simulink model "Katex_FullCar_R2017b_V03"  (R2026a)
settings: Solver=ode1  StopTime=1000  FixedStep=Ts  EnableMultiTasking=on
PostLoadFcn:
  | , if any(exist('dsrtsu_mdlpostloadfcn', 'file') == [2, 3, 6]), try dsrtsu_mdlpostloadfcn('Execute', bdroot); catch fprintf('Error in PostLoadFcn (dsrtsu_mdlpostloadfcn) for model "%s":\n %s\n', bdroot, lasterr); end, end,
  | , if any(exist('dsrtsu_mdlpostloadfcn', 'file') ~= 0), dsrtsu_mdlpostloadfcn('Execute', bdroot); end,
InitFcn:
  | , if any(exist('rtifpga_mdlclblib', 'file') ~= 0), rtifpga_mdlclblib('Init', bdroot); end,
  | 
  | 
  | init
undefined symbols (not defined in the file): locklim_sus, roundN, Ts
libraries: sl_discontinuities x29, simulink_extras x26, simulink x22, mjLib x1
(part 3 of 10)

== system Katex_FullCar_R2017b_V03/DGIST/_High_Level_Ctrl/Chassis_FF_ctrl ==
  note: m/s
  note: Output
      |
      | Load단
      |
      | FL
      | FR
      | RL
      | RR
  note: rad/s
  note: m/s
  note: deg/s
  note: rad/s 여야함
  note: rad/s
  Add1 : Sum  Inputs=+-
  Add3 : Sum
  Divide1 : Product  Inputs=**
  Kinematic_Mapping_FF : MATLAB Function  TreatAsAtomicUnit=on
  Multiply1 : Gain  Gain=pi/180
  Multiply3 : Gain  Gain=180/pi
  Mux : Mux  Inputs=2
  P Control1 : Subsystem
      mask Display: disp('P Control');
  FF_DriveVel_ref : Outport
  FF_SteerPos_ref : Outport  Port=2
  Body_ref_scope : Outport  Port=3
  wires:
  [Body_Vx_ref] -> Kinematic_Mapping_FF/1(Vx_ref)
  [YawRate_FB_ref] -> Kinematic_Mapping_FF/2(YawRate_ref)
  [Wheel_Radius] -> Kinematic_Mapping_FF/5(WheelRadius)
  [Steer_Ref_Limit] -> Kinematic_Mapping_FF/6(SteerLimit)
  Kinematic_Mapping_FF/1(DriveVel_ref) -> FF_DriveVel_ref/1
  Kinematic_Mapping_FF/2(SteerPos_ref) -> FF_SteerPos_ref/1
  [Chassis_wheelbase] -> Kinematic_Mapping_FF/3(L)
  [Chassis_wheelTrack] -> Kinematic_Mapping_FF/4(W)
  Mux/1 -> Body_ref_scope/1
  [Body_Vx_ref] -> Mux/1
  [Body_YawRate_ref] -> Multiply3/1
  Multiply3/1 -> Mux/2
  [Body_YawRate_FB_OnOff] -> Divide1/2
  Divide1/1 -> P Control1/1(err)
  [Body_YawRate_ref] -> Add1/1, Add3/1
  Add3/1 -> [YawRate_FB_ref]
  Multiply1/1 -> Add1/2
  P Control1/1(Out1) -> Add3/2
  Add1/1 -> Divide1/1
  [AngRateYaw_degps] -> Multiply1/1

== system Katex_FullCar_R2017b_V03/DGIST/_High_Level_Ctrl/If Action Subsystem1 ==
  In1 : Inport
  In2 : Inport  Port=2
  In3 : Inport  Port=3
  Action Port : ActionPort  ActionPortLabel=elseif(u1 == 1)
  Out1 : Outport  VectorParamsAs1DForOutWhenUnconnected=off
  Out2 : Outport  Port=2  VectorParamsAs1DForOutWhenUnconnected=off
  Out3 : Outport  Port=3  VectorParamsAs1DForOutWhenUnconnected=off
  wires:
  In1/1 -> Out1/1
  In2/1 -> Out2/1
  In3/1 -> Out3/1

== system Katex_FullCar_R2017b_V03/DGIST/_High_Level_Ctrl/If Action Subsystem5 ==
  In1 : Inport
  In2 : Inport  Port=2
  In3 : Inport  Port=3
  Action Port : ActionPort  ActionPortLabel=if(u1 == 0)
  Out1 : Outport  VectorParamsAs1DForOutWhenUnconnected=off
  Out2 : Outport  Port=2  VectorParamsAs1DForOutWhenUnconnected=off
  Out3 : Outport  Port=3  VectorParamsAs1DForOutWhenUnconnected=off
  wires:
  In1/1 -> Out1/1
  In2/1 -> Out2/1
  In3/1 -> Out3/1

== system Katex_FullCar_R2017b_V03/DGIST/_High_Level_Ctrl/Orientation_Pos_Ctrl ==
  note: deg
  note: rad
  note: Output
      |
      | Suspension Load-side Position (deg)
      |
      | FL
      | FR
      | RL
      | RR
  note: 모터 회전방향 확인 필요(부호 확인 필요)
      |
      | z의 양의 방향을 위쪽으로 정의했다면
      |
      | Load side vel
      | SusVel_ref >0 => 아래로 이동
      | SusVel_ref<0 => 위로 이동
  note: Load deg
  note: deg
  Body_Pitch_PID_ctrl : Subsystem
  Body_Roll_PID_ctrl : Subsystem
  Constant : Constant  Value=180/pi
  Constant4 : Constant  Value=0
  Constant5 : Constant  Value=30
  Demux : Demux  Commented=on
  Divide : Product  Inputs=**
  Gain{,1..6} (7 alike) : Gain  Gain=pi/180
  Goto1 : Goto  Commented=on  GotoTag=SusFR_Load_Pos_Ref  TagVisibility=global
  Goto2 : Goto  Commented=on  GotoTag=SusRL_Load_Pos_Ref  TagVisibility=global
  Goto3 : Goto  Commented=on  GotoTag=SusRR_Load_Pos_Ref  TagVisibility=global
  Goto4 : Goto  Commented=on  GotoTag=SusFL_Load_Pos_Ref  TagVisibility=global
  MATLAB Function : MATLAB Function  TreatAsAtomicUnit=on
  Mux : Mux
  Mux1 : Mux  Inputs=2
  Scope : Scope
      settings: ActiveDisplayYMinimum=-1  ActiveDisplayYMaximum=1  DataLoggingVariableName=ScopeData7
  Out1 : Outport  VectorParamsAs1DForOutWhenUnconnected=off
  Ori_Sus_Load_Pos_Ref : Outport  Port=2
  wires:
  [Chassis_wheelbase] -> MATLAB Function/4(RobotWidth)
  [Chassis_wheelTrack] -> MATLAB Function/5(RobotLength)
  [Sus_Length] -> MATLAB Function/6(SusLinkLength)
  Demux/4 -> Goto3/1
  Demux/3 -> Goto2/1
  Demux/2 -> Goto1/1
  Demux/1 -> Goto4/1
  MATLAB Function/1(SusPos_ref) -> Divide/1
  Constant/1 -> Divide/2
  Mux/1 -> MATLAB Function/3(SusPos_neutral)
  Gain/1 -> MATLAB Function/1(Roll_ref)
  Gain1/1 -> MATLAB Function/2(Pitch_ref)
  Gain2/1 -> Mux/1
  Gain3/1 -> Mux/2
  Gain4/1 -> Mux/3
  Gain5/1 -> Mux/4
  Constant4/1 -> Gain5/1, Gain4/1, Gain3/1, Gain2/1
  Gain6/1 -> MATLAB Function/7(SusPosLimit)
  Constant5/1 -> Gain6/1
  [Body_RollRate_ref] -> Body_Roll_PID_ctrl/1(In1)
  [Body_PitchRate_ref] -> Body_Pitch_PID_ctrl/1(In1)
  Body_Pitch_PID_ctrl/1(Out1) -> Gain1/1
  Body_Roll_PID_ctrl/1(Out1) -> Gain/1
  [AngRoll_deg] -> Body_Roll_PID_ctrl/2(In2)
  [AngPitch_deg] -> Body_Pitch_PID_ctrl/2(In2)
  Mux1/1 -> Out1/1
  [Body_RollRate_ref] -> Mux1/1
  [Body_PitchRate_ref] -> Mux1/2
  Divide/1 -> Scope/1, Ori_Sus_Load_Pos_Ref/1

== system Katex_FullCar_R2017b_V03/DGIST/_High_Level_Ctrl/Orientation_Vel_Ctrl ==
  note: rad/s
  note: Output
      |
      | Suspension Load-side Velocity
      |
      | FL
      | FR
      | RL
      | RR
  note: Sus Load Position 가져와야함
  note: 모터 회전방향 확인 필요(부호 확인 필요)
      |
      | z의 양의 방향을 위쪽으로 정의했다면
      |
      | Load side vel
      | SusVel_ref >0 => 아래로 이동
      | SusVel_ref<0 => 위로 이동
  DOB_Dis : Constant  Value=0
  Demux : Demux
  MATLAB Function : MATLAB Function  TreatAsAtomicUnit=on
  Ts : Constant  Value=Ts
  tag scope: SusFL_Load_Vel_Ref=global, SusFR_Load_Vel_Ref=global, SusRL_Load_Vel_Ref=global, SusRR_Load_Vel_Ref=global
  wires:
  [Body_RollRate_ref] -> MATLAB Function/1(RollRate_ref)
  [Body_PitchRate_ref] -> MATLAB Function/2(PitchRate_ref)
  DOB_Dis/1 -> MATLAB Function/5(disturbance)
  [Chassis_wheelTrack] -> MATLAB Function/7(RobotWidth)
  [Chassis_wheelbase] -> MATLAB Function/8(RobotLength)
  [Sus_LinkLength] -> MATLAB Function/9(SusLinkLength)
  Ts/1 -> MATLAB Function/11(Ts)
  [Ori_DOB_CutOff] -> MATLAB Function/10(DOB_cutoff_freq)
  [Ori_DOB_OnOff] -> MATLAB Function/12(DOB_onoff)
  MATLAB Function/1(SusVel_ref) -> Demux/1
  Demux/4 -> [SusRR_Load_Vel_Ref]
  Demux/3 -> [SusRL_Load_Vel_Ref]
  Demux/2 -> [SusFR_Load_Vel_Ref]
  Demux/1 -> [SusFL_Load_Vel_Ref]

== system Katex_FullCar_R2017b_V03/DGIST/_Low_Level_Ctrl/Driving_Low_Level_Controller ==
  note: Motor Input 4X1
  note: Target Torque
  note: Output
      |
      | 1: Motor angular velocity (단위가 RPM 이여야함)
      | 2: Motor Torque (단위가 Target Torque 여야함)
      | 3: 전륜 RPM / 후륜 Target Torque 0 이여야함
      |
      | 각 Box Output에 input mode도 같이 나와야함 4X1로 나와야함
      | (8: position / 9: Velocity / 10: Torque)
  note: 0: Pos Mode(안씀)
      | 1: Vel Mode
      | 2: Torque Mode
      | 3: FB(전륜 Vel Mode, 후륜 Torque Mode)
  note: Motor Input Mode
  note: Motor Input Mode
  note: 전륜: RPM/ 후륜: Target Torque 0
  note: Motor Input Mode
  note: Load m/s
  In1 : Inport
  Demux : Demux
  Divide1 : Product  Inputs=**
  FB Mode : Subsystem  TreatAsAtomicUnit=on
  If1 : If  IfExpression=u1 == 1  ElseIfExpressions=u1 == 2,u1 == 3
  Merge1 : Merge  Inputs=3
  Merge2 : Merge  Inputs=3
  Torque Mode : Subsystem  TreatAsAtomicUnit=on
  Tunning reference box : Subsystem
  Velocity Mode : Subsystem  TreatAsAtomicUnit=on
  Out1 : Outport
  tag scope: DriFL_Motor_OperationMode=global, DriFR_Motor_OperationMode=global, DriRL_Motor_OperationMode=global, DriRR_Motor_OperationMode=global
  wires:
  If1/1 -> Velocity Mode/Action
  If1/2 -> Torque Mode/Action
  [ctrl_onoff] -> Divide1/1
  [Dri_Motor_Mode] -> If1/1
  Demux/1 -> [DriFL_Motor_OperationMode]
  Merge2/1 -> Demux/1
  Demux/4 -> [DriRR_Motor_OperationMode]
  Velocity Mode/1(Out1) -> Merge1/1
  Velocity Mode/2(Out2) -> Merge2/1
  Demux/2 -> [DriFR_Motor_OperationMode]
  If1/3 -> FB Mode/Action
  Merge1/1 -> Divide1/2
  Demux/3 -> [DriRL_Motor_OperationMode]
  [Dri_Vel] -> FB Mode/1(In1)
  In1/1 -> [Dri_Vel]
  Divide1/1 -> Out1/1
  [Dri_Vel] -> Velocity Mode/1(In1)
  FB Mode/1(Out1) -> Merge1/3
  Torque Mode/1(Out1) -> Merge1/2
  FB Mode/2(Out2) -> Merge2/3
  Torque Mode/2(Out2) -> Merge2/2

== system Katex_FullCar_R2017b_V03/DGIST/_Low_Level_Ctrl/Steering_Low_Level_Controller ==
  note: Motor Input 4X1
  note: Motor Input Mode
  note: Target Torque
  note: Motor Input Mode
  note: 0: Pos Mode
      | 1: Vel Mode(안씀)
      | 2: Torque Mode
      | 3: FB(Pos Mode)
  note: Output
      |
      | 0: Motor angular Position (단위 cnt)
      | 1: Motor angular velocity (안씀)
      | 2: Motor Target Torque (Target Torque)
      |
      | 각 Box Output에 input mode도 같이 나와야함 4X1로 나와야함
      | (8: position / 9: Velocity / 10: Torque)
  note: cnt
  note: cnt
  In1 : Inport
  Constant : Constant  Value=0
  Demux : Demux
  Divide1 : Product  Inputs=**
  Gain : Gain
  If1 : If  IfExpression=u1 == 0  ElseIfExpressions=u1 == 2
  Merge : Merge
  Merge1 : Merge
  Mux : Mux
  Position Mode : Subsystem  TreatAsAtomicUnit=on
  Sine Wave : Sin  Amplitude=10  Frequency=0.2  SampleTime=0
  Torque Mode : Subsystem  TreatAsAtomicUnit=on
  Out1 : Outport
  tag scope: StrFL_Motor_OperationMode=global, StrFR_Motor_OperationMode=global, StrRL_Motor_OperationMode=global, StrRR_Motor_OperationMode=global
  wires:
  If1/1 -> Position Mode/Action
  If1/2 -> Torque Mode/Action
  [ctrl_onoff] -> Divide1/1
  Divide1/1 -> Out1/1
  [Str_Motor_Mode] -> If1/1
  Demux/1 -> [StrFL_Motor_OperationMode]
  Demux/4 -> [StrRR_Motor_OperationMode]
  Demux/2 -> [StrFR_Motor_OperationMode]
  Demux/3 -> [StrRL_Motor_OperationMode]
  In1/1 -> [Str_Load_Pos_Ref]
  Mux/1 -> Position Mode/1(In1)
  Gain/1 -> Mux/2, Mux/3, Mux/4, Mux/1
  Constant/1 -> Gain/1
  Torque Mode/1(Out1) -> Merge/2
  Merge/1 -> Divide1/2
  Position Mode/1(Out1) -> Merge/1
  Merge1/1 -> Demux/1
  Position Mode/2(Out2) -> Merge1/1
  Torque Mode/2(Out2) -> Merge1/2

== system Katex_FullCar_R2017b_V03/DGIST/_Low_Level_Ctrl/Suspension_Low_Level_Controller ==
  note: 추가해야 할 부분(Sus control부분에서)
      | Position Mapping 입력부분 RollRate,PitchRate 같이 사용하는 중 (High level)
      | SusPosLimit 연결 필요(High level)
      | Velocity DOB 입력 미연결 상태 IMU, SusPos_act 연결필요
      | DOB disturbance check 부분 4X1로 만들어야 할 필요 있음
  note: Motor Input 4X1
  note: Target Torque
  note: 0: Pos Mode
      | 1: Vel Mode
      | 2: Torque Mode
  note: Motor Input Mode
  note: RPM
  note: Motor Input Mode
  note: Motor Input Mode
  note: 0: Pos Mode
      | 1: Vel Mode
      | 2: Torque Mode (안씀)
      | 3: FB(전륜 Vel Mode, 후륜 Torque Mode) (안씀)
  note: Output
      |
      | 0: Motor angular Position (단위 cnt)
      | 1: Motor angular velocity (단위 RPM)
      | 2: Motor Target Torque (안씀)
      |
      | 각 Box Output에 input mode도 같이 나와야함 4X1로 나와야함
      | (8: position / 9: Velocity / 10: Torque)
  note: cnt
  note: Load deg
  In1 : Inport
  Demux : Demux
  Divide1 : Product  Inputs=**
  If1 : If  IfExpression=u1 == 0  ElseIfExpressions=u1 == 1,u1 == 2
  Merge : Merge  Inputs=3
  Merge1 : Merge  Inputs=3
  Position Mode : Subsystem  TreatAsAtomicUnit=on
  Torque Mode : Subsystem  TreatAsAtomicUnit=on
  Tunning reference box : Subsystem
  Velocity Mode : Subsystem  TreatAsAtomicUnit=on
  Out1 : Outport
  tag scope: SusFL_Motor_OperationMode=global, SusFR_Motor_OperationMode=global, SusRL_Motor_OperationMode=global, SusRR_Motor_OperationMode=global
  wires:
  If1/1 -> Position Mode/Action
  If1/2 -> Velocity Mode/Action
  [ctrl_onoff] -> Divide1/1
  [Sus_Motor_Mode] -> If1/1
  Demux/1 -> [SusFL_Motor_OperationMode]
  Demux/4 -> [SusRR_Motor_OperationMode]
  Demux/2 -> [SusFR_Motor_OperationMode]
  If1/3 -> Torque Mode/Action
  Demux/3 -> [SusRL_Motor_OperationMode]
  [Sus_Load_Deg_Limit] -> Position Mode/2(In2)
  [Sus_Load_Pos_Ref] -> Position Mode/1(In1)
  Merge/1 -> Demux/1
  Position Mode/2(Out2) -> Merge/1
  Velocity Mode/2(Out2) -> Merge/2
  Torque Mode/2(Out2) -> Merge/3
  Merge1/1 -> Divide1/2
  Position Mode/1(Out1) -> Merge1/1
  Velocity Mode/1(Out1) -> Merge1/2
  [Sus_Torque_Limit] -> Torque Mode/2(In2)
  In1/1 -> [Sus_Load_Pos_Ref]
  Torque Mode/1(Out1) -> Merge1/3
  [Sus_Load_Pos_Ref] -> Torque Mode/1(In1)
  Divide1/1 -> Out1/1

== system Katex_FullCar_R2017b_V03/DGIST/_Reference_Generator/If Action Subsystem1 ==
  In1 : Inport
  Action Port : ActionPort  ActionPortLabel=elseif(u1 == 2)
  Out1 : Outport  VectorParamsAs1DForOutWhenUnconnected=off
  wires:
  In1/1 -> Out1/1

== system Katex_FullCar_R2017b_V03/DGIST/_Reference_Generator/If Action Subsystem2 ==
  In1 : Inport
  Action Port : ActionPort  ActionPortLabel=elseif(u1 == 3)
  Demux : Demux
  Scope : Scope
      settings: DataLoggingVariableName=ScopeData2
  Terminator : Terminator
  Terminator1 : Terminator
  Terminator2 : Terminator
  Out1 : Outport  VectorParamsAs1DForOutWhenUnconnected=off
  wires:
  In1/1 -> Demux/1, Out1/1
  Demux/3 -> Scope/1
  Demux/1 -> Terminator/1
  Demux/2 -> Terminator1/1
  Demux/4 -> Terminator2/1

== system Katex_FullCar_R2017b_V03/DGIST/_Reference_Generator/If Action Subsystem3 ==
  In1 : Inport
  Action Port : ActionPort  ActionPortLabel=else
  Out1 : Outport  VectorParamsAs1DForOutWhenUnconnected=off
  wires:
  In1/1 -> Out1/1

== system Katex_FullCar_R2017b_V03/DGIST/_Reference_Generator/If Action Subsystem4 ==
  In1 : Inport
  Action Port : ActionPort  ActionPortLabel=if(u1 == 1)
  Out1 : Outport  VectorParamsAs1DForOutWhenUnconnected=off
  wires:
  In1/1 -> Out1/1

== system Katex_FullCar_R2017b_V03/DGIST/_Reference_Generator/Orientation Profile ==
  note: output
      |
      | Vx
      | gamma
      | RollRate
      | PitchRate
  Compare To Constant1 : simulink/Logic and Bit Operations/Compare To Constant  relop===  const=3  OutDataTypeStr=boolean
  Compare To Constant2 : simulink/Logic and Bit Operations/Compare To Constant  relop===  const=3  OutDataTypeStr=boolean
  Constant : Constant  Value=0
  Data Type Conversion1 : DataTypeConversion  OutDataTypeStr=double  SaturateOnIntegerOverflow=off  RndMeth=Floor
  Data Type Conversion2 : DataTypeConversion  OutDataTypeStr=double  SaturateOnIntegerOverflow=off  RndMeth=Floor
  Divide1 : Product  Inputs=**
  Divide2 : Product  Inputs=**
  MATLAB Function : MATLAB Function  TreatAsAtomicUnit=on
  MATLAB Function1 : MATLAB Function  TreatAsAtomicUnit=on
  Output : Mux
  Ref3_Output : Outport
  wires:
  Output/1 -> Ref3_Output/1
  Constant/1 -> Output/2, Output/1
  [Local_Time] -> MATLAB Function/1(t)
  Divide2/1 -> MATLAB Function/4(flag)
  [RollRate_freq_ref_cmd] -> MATLAB Function/2(f)
  [RollRate_mag_ref_cmd] -> MATLAB Function/3(mag)
  [Local_Time] -> MATLAB Function1/1(t)
  Divide1/1 -> MATLAB Function1/4(flag)
  [PitchRate_freq_ref_cmd] -> MATLAB Function1/2(f)
  [PitchRate_mag_ref_cmd] -> MATLAB Function1/3(mag)
  MATLAB Function/1(y) -> Output/3
  MATLAB Function1/1(y) -> Output/4
  Compare To Constant1/1 -> Data Type Conversion1/1
  Data Type Conversion1/1 -> Divide2/2
  [ctrl_onoff] -> Divide2/1
  [Scenario_cmd] -> Compare To Constant1/1
  [ctrl_onoff] -> Divide1/1
  Data Type Conversion2/1 -> Divide1/2
  [Scenario_cmd] -> Compare To Constant2/1
  Compare To Constant2/1 -> Data Type Conversion2/1

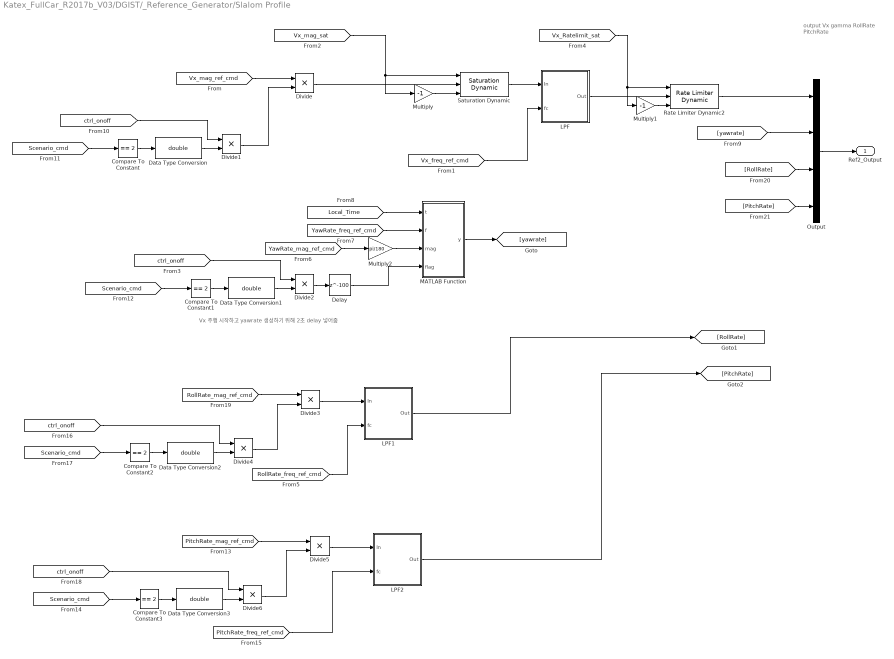
== system Katex_FullCar_R2017b_V03/DGIST/_Reference_Generator/Slalom Profile ==
  note: Vx 주행 시작하고 yawrate 생성하기 위해 2초 delay 넣어줌
  note: output
      |
      | Vx
      | gamma
      | RollRate
      | PitchRate
  Compare To Constant{,1..3} (4 alike) : simulink/Logic and Bit Operations/Compare To Constant  relop===  const=2  OutDataTypeStr=boolean
  Data Type Conversion{,1..3} (4 alike) : DataTypeConversion  OutDataTypeStr=double  SaturateOnIntegerOverflow=off  RndMeth=Floor
  Delay : Delay  DelayLength=100
  Divide{,1..6} (7 alike) : Product  Inputs=**
  LPF : Subsystem
  LPF1 : Subsystem
  LPF2 : Subsystem
  MATLAB Function : MATLAB Function  TreatAsAtomicUnit=on
  Multiply : Gain  Gain=-1
  Multiply1 : Gain  Gain=-1
  Multiply2 : Gain  Gain=pi/180
  Output : Mux
  Rate Limiter Dynamic2 : sl_discontinuities/Rate Limiter Dynamic
  Saturation Dynamic : sl_discontinuities/Saturation Dynamic  OutMin=[]  OutMax=[]  OutDataTypeStr=Inherit: Same as second input  OutDataType=fixdt(1, 16)  OutScaling=2^-10  DoSatur=off
  Ref2_Output : Outport
  wires:
  Multiply/1 -> Saturation Dynamic/3
  Output/1 -> Ref2_Output/1
  [Vx_mag_sat] -> Multiply/1, Saturation Dynamic/1
  Divide/1 -> Saturation Dynamic/2
  Rate Limiter Dynamic2/1 -> Output/1
  [Vx_Ratelimit_sat] -> Multiply1/1, Rate Limiter Dynamic2/1
  Multiply1/1 -> Rate Limiter Dynamic2/3
  [Vx_freq_ref_cmd] -> LPF/2(fc)
  Saturation Dynamic/1 -> LPF/1(In)
  [Vx_mag_ref_cmd] -> Divide/1
  LPF/1(Out) -> Rate Limiter Dynamic2/2
  Divide1/1 -> Divide/2
  Divide2/1 -> Delay/1
  [Local_Time] -> MATLAB Function/1(t)
  [YawRate_freq_ref_cmd] -> MATLAB Function/2(f)
  [YawRate_mag_ref_cmd] -> Multiply2/1
  MATLAB Function/1(y) -> [yawrate]
  [yawrate] -> Output/2
  [ctrl_onoff] -> Divide1/1
  [Scenario_cmd] -> Compare To Constant/1
  Data Type Conversion/1 -> Divide1/2
  Compare To Constant/1 -> Data Type Conversion/1
  [ctrl_onoff] -> Divide2/1
  [Scenario_cmd] -> Compare To Constant1/1
  Data Type Conversion1/1 -> Divide2/2
  Compare To Constant1/1 -> Data Type Conversion1/1
  Delay/1 -> MATLAB Function/4(flag)
  Multiply2/1 -> MATLAB Function/3(mag)
  [RollRate_mag_ref_cmd] -> Divide3/1
  [Scenario_cmd] -> Compare To Constant3/1
  [ctrl_onoff] -> Divide6/1
  Divide3/1 -> LPF1/1(In)
  Divide6/1 -> Divide5/2
  Compare To Constant3/1 -> Data Type Conversion3/1
  Data Type Conversion2/1 -> Divide4/2
  Compare To Constant2/1 -> Data Type Conversion2/1
  [ctrl_onoff] -> Divide4/1
  Divide4/1 -> Divide3/2
  LPF2/1(Out) -> [PitchRate]
  Divide5/1 -> LPF2/1(In)
  Data Type Conversion3/1 -> Divide6/2
  LPF1/1(Out) -> [RollRate]
  [Scenario_cmd] -> Compare To Constant2/1
  [RollRate_freq_ref_cmd] -> LPF1/2(fc)
  [RollRate] -> Output/3
  [PitchRate] -> Output/4
  [PitchRate_mag_ref_cmd] -> Divide5/1
  [PitchRate_freq_ref_cmd] -> LPF2/2(fc)

== system Katex_FullCar_R2017b_V03/DGIST/_Reference_Generator/Straight Profile ==
  note: m/s
  note: output
      |
      | Vx
      | gamma
      | RollRate
      | PitchRate
  Compare To Constant : simulink/Logic and Bit Operations/Compare To Constant  relop===  const=1  OutDataTypeStr=boolean
  Compare To Constant1 : simulink/Logic and Bit Operations/Compare To Constant  relop===  const=1  OutDataTypeStr=boolean
  Compare To Constant2 : simulink/Logic and Bit Operations/Compare To Constant  relop===  const=1  OutDataTypeStr=boolean
  Constant : Constant  Value=0
  Data Type Conversion : DataTypeConversion  OutDataTypeStr=double  SaturateOnIntegerOverflow=off  RndMeth=Floor
  Data Type Conversion1 : DataTypeConversion  OutDataTypeStr=double  SaturateOnIntegerOverflow=off  RndMeth=Floor
  Data Type Conversion2 : DataTypeConversion  OutDataTypeStr=double  SaturateOnIntegerOverflow=off  RndMeth=Floor
  Divide{,1..5} (6 alike) : Product  Inputs=**
  LPF : Subsystem
  LPF1 : Subsystem
  LPF2 : Subsystem
  Multiply : Gain  Gain=-1
  Multiply1 : Gain  Gain=-1
  Output : Mux
  Rate Limiter Dynamic2 : sl_discontinuities/Rate Limiter Dynamic
  Saturation Dynamic : sl_discontinuities/Saturation Dynamic  OutMin=[]  OutMax=[]  OutDataTypeStr=Inherit: Same as second input  OutDataType=fixdt(1, 16)  OutScaling=2^-10  DoSatur=off
  Ref1_Output : Outport
  wires:
  [Vx_mag_ref_cmd] -> Divide/1
  Divide/1 -> Saturation Dynamic/2
  Saturation Dynamic/1 -> LPF/1(In)
  [Vx_freq_ref_cmd] -> LPF/2(fc)
  LPF/1(Out) -> Rate Limiter Dynamic2/2
  Rate Limiter Dynamic2/1 -> Output/1
  Constant/1 -> Output/2
  Output/1 -> Ref1_Output/1
  [Vx_mag_sat] -> Multiply/1, Saturation Dynamic/1
  Multiply/1 -> Saturation Dynamic/3
  [Vx_Ratelimit_sat] -> Multiply1/1, Rate Limiter Dynamic2/1
  Multiply1/1 -> Rate Limiter Dynamic2/3
  [Scenario_cmd] -> Compare To Constant/1
  Compare To Constant/1 -> Data Type Conversion/1
  [ctrl_onoff] -> Divide1/1
  Divide1/1 -> Divide/2
  Data Type Conversion/1 -> Divide1/2
  [Scenario_cmd] -> Compare To Constant1/1
  Data Type Conversion1/1 -> Divide3/2
  Compare To Constant1/1 -> Data Type Conversion1/1
  [ctrl_onoff] -> Divide3/1
  Divide3/1 -> Divide2/2
  [RollRate_mag_ref_cmd] -> Divide2/1
  Divide2/1 -> LPF1/1(In)
  [RollRate_freq_ref_cmd] -> LPF1/2(fc)
  LPF1/1(Out) -> Output/3
  Data Type Conversion2/1 -> Divide5/2
  Compare To Constant2/1 -> Data Type Conversion2/1
  [ctrl_onoff] -> Divide5/1
  Divide5/1 -> Divide4/2
  [Scenario_cmd] -> Compare To Constant2/1
  Divide4/1 -> LPF2/1(In)
  LPF2/1(Out) -> Output/4
  [PitchRate_freq_ref_cmd] -> LPF2/2(fc)
  [PitchRate_mag_ref_cmd] -> Divide4/1

== system Katex_FullCar_R2017b_V03/Locomotion/Conditioning/Driving mode ==
  cmd : Inport
  mode : Inport  Port=2
  Compare To Constant : simulink/Logic and Bit Operations/Compare To Constant  relop===  const=4  OutDataTypeStr=boolean
  Constant1 : Constant  Value=-1
  Constant2 : Constant
  Demux : Demux
  Gain : Gain
  Gain1 : Gain
  Multiply : Product
  Multiply1 : Product
  Mux : Mux
  Sat : Saturate  UpperLimit=1.5  LowerLimit=-1.5
  Switch : Switch  Criteria=u2 > Threshold  SaturateOnIntegerOverflow=off  InputSameDT=off
  cmd_out : Outport  VectorParamsAs1DForOutWhenUnconnected=off
  wires:
  Compare To Constant/1 -> Switch/2
  Constant2/1 -> Switch/3
  Constant1/1 -> Switch/1
  Switch/1 -> [sign_FLRR]
  mode/1 -> Compare To Constant/1
  [sign_FLRR] -> Multiply/1
  Gain/1 -> Mux/2  "FR_velref_mps"
  Gain1/1 -> Mux/4  "RR_velref_mps"
  [sign_FLRR] -> Multiply1/1
  Mux/1 -> Sat/1
  Multiply/1 -> Mux/1  "FL_velref_mps"
  Multiply1/1 -> Mux/3  "RL_velref_mps"
  Sat/1 -> cmd_out/1  "dev_velref_mps"
  Demux/1 -> Multiply/2
  Demux/2 -> Gain/1
  Demux/3 -> Multiply1/2
  Demux/4 -> Gain1/1
  cmd/1 -> Demux/1

== system Katex_FullCar_R2017b_V03/Locomotion/Conditioning/Drv_LPF ==
  note: s = 2/Ts*(z-1)/(z+1)
  note: H(s) = 1/(tau*s+1)
  note: y(n) = [Ts*{x(n)+x(n-1)}+(2*tau-Ts)*y(n-1)]/(2*tau+Ts)
  note: LPF : tau = 1/(2*pi*fc)
  In : Inport
  fc : Inport  Port=2
  Constant : Constant  Value=Ts  SampleTime=Ts
  Constant1 : Constant  SampleTime=Ts
  Product1 : Product  Inputs=*/  RndMeth=Zero
  Product11 : Product  RndMeth=Zero
  Product2 : Product  Inputs=*/  RndMeth=Zero
  Sum1 : Sum  Inputs=+-  InputSameDT=on  SaturateOnIntegerOverflow=on  OutDataTypeStr=Inherit: Same as first input
  Sum2 : Sum  InputSameDT=on  SaturateOnIntegerOverflow=on  OutDataTypeStr=Inherit: Same as first input
  Sum3 : Sum  InputSameDT=on  SaturateOnIntegerOverflow=on  OutDataTypeStr=Inherit: Same as first input
  Sum4 : Sum  InputSameDT=on  SaturateOnIntegerOverflow=on  OutDataTypeStr=Inherit: Same as first input
  d : UnitDelay  SampleTime=Ts
  d1 : UnitDelay  SampleTime=Ts
  gain : Gain  Gain=Ts  SaturateOnIntegerOverflow=on  OutDataTypeStr=Inherit: Same as input  ParamDataTypeStr=Inherit: Same as input
  gain1 : Gain  Gain=2  SaturateOnIntegerOverflow=on  OutDataTypeStr=Inherit: Same as input  ParamDataTypeStr=Inherit: Same as input
  gain2 : Gain  Gain=2*pi  SaturateOnIntegerOverflow=on  OutDataTypeStr=Inherit: Same as input  ParamDataTypeStr=Inherit: Same as input
  Out : Outport
  wires:
  gain2/1 -> Product2/2
  Constant1/1 -> Product2/1
  Product2/1 -> gain1/1
  Product1/1 -> d/1, Out/1
  Sum4/1 -> Product1/2
  Sum2/1 -> Product1/1
  d/1 -> Product11/2
  gain1/1 -> Sum4/1, Sum1/1
  fc/1 -> gain2/1
  Constant/1 -> Sum4/2, Sum1/2
  Sum1/1 -> Product11/1
  Product11/1 -> Sum2/2
  gain/1 -> Sum2/1
  Sum3/1 -> gain/1
  d1/1 -> Sum3/2
  In/1 -> d1/1, Sum3/1

== system Katex_FullCar_R2017b_V03/Locomotion/Conditioning/Drv_LPF1 ==
  note: LPF : tau = 1/(2*pi*fc)
  note: y(n) = [Ts*{x(n)+x(n-1)}+(2*tau-Ts)*y(n-1)]/(2*tau+Ts)
  note: H(s) = 1/(tau*s+1)
  note: s = 2/Ts*(z-1)/(z+1)
  In : Inport
  fc : Inport  Port=2
  Constant : Constant  Value=Ts  SampleTime=Ts
  Constant1 : Constant  SampleTime=Ts
  Product1 : Product  Inputs=*/  RndMeth=Zero
  Product11 : Product  RndMeth=Zero
  Product2 : Product  Inputs=*/  RndMeth=Zero
  Sum1 : Sum  Inputs=+-  InputSameDT=on  SaturateOnIntegerOverflow=on  OutDataTypeStr=Inherit: Same as first input
  Sum2 : Sum  InputSameDT=on  SaturateOnIntegerOverflow=on  OutDataTypeStr=Inherit: Same as first input
  Sum3 : Sum  InputSameDT=on  SaturateOnIntegerOverflow=on  OutDataTypeStr=Inherit: Same as first input
  Sum4 : Sum  InputSameDT=on  SaturateOnIntegerOverflow=on  OutDataTypeStr=Inherit: Same as first input
  d : UnitDelay  SampleTime=Ts
  d1 : UnitDelay  SampleTime=Ts
  gain : Gain  Gain=Ts  SaturateOnIntegerOverflow=on  OutDataTypeStr=Inherit: Same as input  ParamDataTypeStr=Inherit: Same as input
  gain1 : Gain  Gain=2  SaturateOnIntegerOverflow=on  OutDataTypeStr=Inherit: Same as input  ParamDataTypeStr=Inherit: Same as input
  gain2 : Gain  Gain=2*pi  SaturateOnIntegerOverflow=on  OutDataTypeStr=Inherit: Same as input  ParamDataTypeStr=Inherit: Same as input
  Out : Outport
  wires:
  In/1 -> Sum3/1, d1/1
  d1/1 -> Sum3/2
  Sum3/1 -> gain/1
  gain/1 -> Sum2/1
  Product11/1 -> Sum2/2
  Sum1/1 -> Product11/1
  Constant/1 -> Sum1/2, Sum4/2
  fc/1 -> gain2/1
  gain1/1 -> Sum1/1, Sum4/1
  d/1 -> Product11/2
  Sum2/1 -> Product1/1
  Sum4/1 -> Product1/2
  Product1/1 -> Out/1, d/1
  Product2/1 -> gain1/1
  Constant1/1 -> Product2/1
  gain2/1 -> Product2/2

== system Katex_FullCar_R2017b_V03/Locomotion/Conditioning/Drv_LPF2 ==
  note: s = 2/Ts*(z-1)/(z+1)
  note: H(s) = 1/(tau*s+1)
  note: y(n) = [Ts*{x(n)+x(n-1)}+(2*tau-Ts)*y(n-1)]/(2*tau+Ts)
  note: LPF : tau = 1/(2*pi*fc)
  In : Inport
  fc : Inport  Port=2
  Constant : Constant  Value=Ts  SampleTime=Ts
  Constant1 : Constant  SampleTime=Ts
  Product1 : Product  Inputs=*/  RndMeth=Zero
  Product11 : Product  RndMeth=Zero
  Product2 : Product  Inputs=*/  RndMeth=Zero
  Sum1 : Sum  Inputs=+-  InputSameDT=on  SaturateOnIntegerOverflow=on  OutDataTypeStr=Inherit: Same as first input
  Sum2 : Sum  InputSameDT=on  SaturateOnIntegerOverflow=on  OutDataTypeStr=Inherit: Same as first input
  Sum3 : Sum  InputSameDT=on  SaturateOnIntegerOverflow=on  OutDataTypeStr=Inherit: Same as first input
  Sum4 : Sum  InputSameDT=on  SaturateOnIntegerOverflow=on  OutDataTypeStr=Inherit: Same as first input
  d : UnitDelay  SampleTime=Ts
  d1 : UnitDelay  SampleTime=Ts
  gain : Gain  Gain=Ts  SaturateOnIntegerOverflow=on  OutDataTypeStr=Inherit: Same as input  ParamDataTypeStr=Inherit: Same as input
  gain1 : Gain  Gain=2  SaturateOnIntegerOverflow=on  OutDataTypeStr=Inherit: Same as input  ParamDataTypeStr=Inherit: Same as input
  gain2 : Gain  Gain=2*pi  SaturateOnIntegerOverflow=on  OutDataTypeStr=Inherit: Same as input  ParamDataTypeStr=Inherit: Same as input
  Out : Outport
  wires:
  gain2/1 -> Product2/2
  Constant1/1 -> Product2/1
  Product2/1 -> gain1/1
  Product1/1 -> d/1, Out/1
  Sum4/1 -> Product1/2
  Sum2/1 -> Product1/1
  d/1 -> Product11/2
  gain1/1 -> Sum4/1, Sum1/1
  fc/1 -> gain2/1
  Constant/1 -> Sum4/2, Sum1/2
  Sum1/1 -> Product11/1
  Product11/1 -> Sum2/2
  gain/1 -> Sum2/1
  Sum3/1 -> gain/1
  d1/1 -> Sum3/2
  In/1 -> d1/1, Sum3/1

== system Katex_FullCar_R2017b_V03/Locomotion/Conditioning/Drv_LPF3 ==
  note: LPF : tau = 1/(2*pi*fc)
  note: y(n) = [Ts*{x(n)+x(n-1)}+(2*tau-Ts)*y(n-1)]/(2*tau+Ts)
  note: H(s) = 1/(tau*s+1)
  note: s = 2/Ts*(z-1)/(z+1)
  In : Inport
  fc : Inport  Port=2
  Constant : Constant  Value=Ts  SampleTime=Ts
  Constant1 : Constant  SampleTime=Ts
  Product1 : Product  Inputs=*/  RndMeth=Zero
  Product11 : Product  RndMeth=Zero
  Product2 : Product  Inputs=*/  RndMeth=Zero
  Sum1 : Sum  Inputs=+-  InputSameDT=on  SaturateOnIntegerOverflow=on  OutDataTypeStr=Inherit: Same as first input
  Sum2 : Sum  InputSameDT=on  SaturateOnIntegerOverflow=on  OutDataTypeStr=Inherit: Same as first input
  Sum3 : Sum  InputSameDT=on  SaturateOnIntegerOverflow=on  OutDataTypeStr=Inherit: Same as first input
  Sum4 : Sum  InputSameDT=on  SaturateOnIntegerOverflow=on  OutDataTypeStr=Inherit: Same as first input
  d : UnitDelay  SampleTime=Ts
  d1 : UnitDelay  SampleTime=Ts
  gain : Gain  Gain=Ts  SaturateOnIntegerOverflow=on  OutDataTypeStr=Inherit: Same as input  ParamDataTypeStr=Inherit: Same as input
  gain1 : Gain  Gain=2  SaturateOnIntegerOverflow=on  OutDataTypeStr=Inherit: Same as input  ParamDataTypeStr=Inherit: Same as input
  gain2 : Gain  Gain=2*pi  SaturateOnIntegerOverflow=on  OutDataTypeStr=Inherit: Same as input  ParamDataTypeStr=Inherit: Same as input
  Out : Outport
  wires:
  In/1 -> Sum3/1, d1/1
  d1/1 -> Sum3/2
  Sum3/1 -> gain/1
  gain/1 -> Sum2/1
  Product11/1 -> Sum2/2
  Sum1/1 -> Product11/1
  Constant/1 -> Sum1/2, Sum4/2
  fc/1 -> gain2/1
  gain1/1 -> Sum1/1, Sum4/1
  d/1 -> Product11/2
  Sum2/1 -> Product1/1
  Sum4/1 -> Product1/2
  Product1/1 -> Out/1, d/1
  Product2/1 -> gain1/1
  Constant1/1 -> Product2/1
  gain2/1 -> Product2/2

== system Katex_FullCar_R2017b_V03/Locomotion/Conditioning/Point_Round1 ==
  u : Inport
  N : Inport  Port=2
  Divide : Product  Inputs=*/
  Math Function : Math  Operator=10^u  SignedPower=on
  Multiply : Product
  Round : Rounding  Operator=round
  y : Outport  VectorParamsAs1DForOutWhenUnconnected=off
  wires:
  Divide/1 -> y/1
  Round/1 -> Divide/1
  Multiply/1 -> Round/1
  Math Function/1 -> Divide/2, Multiply/2
  N/1 -> Math Function/1
  u/1 -> Multiply/1

== system Katex_FullCar_R2017b_V03/Locomotion/Conditioning/Point_Round3 ==
  u : Inport
  N : Inport  Port=2
  Divide : Product  Inputs=*/
  Math Function : Math  Operator=10^u  SignedPower=on
  Multiply : Product
  Round : Rounding  Operator=round
  y : Outport  VectorParamsAs1DForOutWhenUnconnected=off
  wires:
  u/1 -> Multiply/1
  N/1 -> Math Function/1
  Math Function/1 -> Multiply/2, Divide/2
  Multiply/1 -> Round/1
  Round/1 -> Divide/1
  Divide/1 -> y/1

== system Katex_FullCar_R2017b_V03/Locomotion/Conditioning/Point_Round4 ==
  u : Inport
  N : Inport  Port=2
  Divide : Product  Inputs=*/
  Math Function : Math  Operator=10^u  SignedPower=on
  Multiply : Product
  Round : Rounding  Operator=round
  y : Outport  VectorParamsAs1DForOutWhenUnconnected=off
  wires:
  Divide/1 -> y/1
  Round/1 -> Divide/1
  Multiply/1 -> Round/1
  Math Function/1 -> Divide/2, Multiply/2
  N/1 -> Math Function/1
  u/1 -> Multiply/1

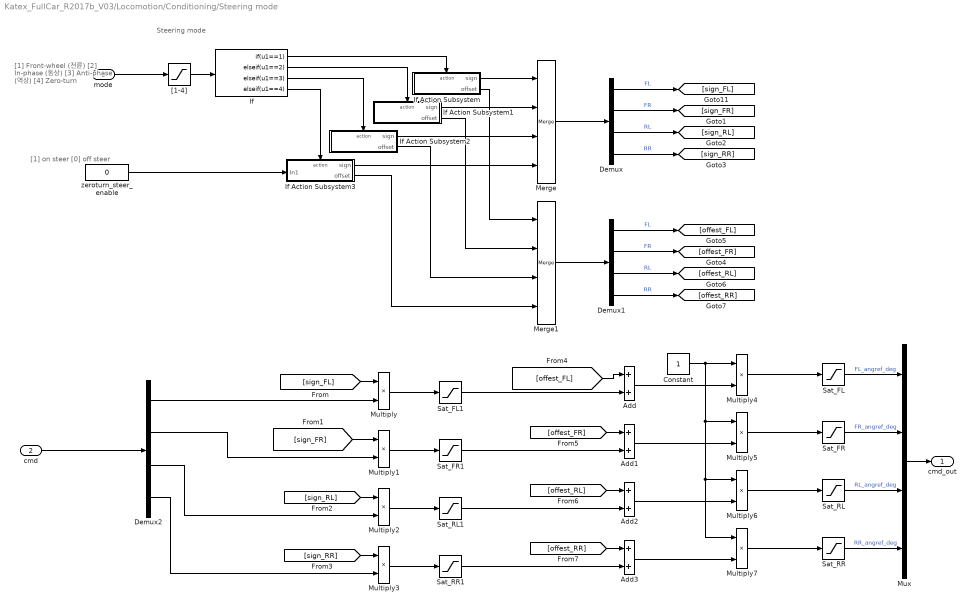
== system Katex_FullCar_R2017b_V03/Locomotion/Conditioning/Steering mode ==
  note: Steering mode
  note: [1] Front-wheel (전륜)
      | [2] In-phase (동상)
      | [3] Anti-phase (역상)
      | [4] Zero-turn
  note: [1] on steer
      | [0] off steer
  mode : Inport
  cmd : Inport  Port=2
  Add{,1..3} (4 alike) : Sum
  Constant : Constant
  Demux : Demux
  Demux1 : Demux
  Demux2 : Demux
  If : If  IfExpression=u1==1  ElseIfExpressions=u1==2,u1==3,u1==4  ShowElse=off
  If Action Subsystem : Subsystem  TreatAsAtomicUnit=on
  If Action Subsystem1 : Subsystem  TreatAsAtomicUnit=on
  If Action Subsystem2 : Subsystem  TreatAsAtomicUnit=on
  If Action Subsystem3 : Subsystem  TreatAsAtomicUnit=on
  Merge : Merge  Inputs=4
  Merge1 : Merge  Inputs=4
  Multiply{,1..7} (8 alike) : Product
  Mux : Mux
  Sat_FL : Saturate  UpperLimit=30  LowerLimit=-50
  Sat_FL1 : Saturate  UpperLimit=30  LowerLimit=-30
  Sat_FR : Saturate  UpperLimit=50  LowerLimit=-30
  Sat_FR1 : Saturate  UpperLimit=30  LowerLimit=-30
  Sat_RL : Saturate  UpperLimit=50  LowerLimit=-30
  Sat_RL1 : Saturate  UpperLimit=30  LowerLimit=-30
  Sat_RR : Saturate  UpperLimit=30  LowerLimit=-50
  Sat_RR1 : Saturate  UpperLimit=30  LowerLimit=-30
  "[1-4]" : Saturate  UpperLimit=4  LowerLimit=1
  zeroturn_steer_enable : Constant  Value=0  SampleTime=Ts
  cmd_out : Outport  VectorParamsAs1DForOutWhenUnconnected=off
  wires:
  Demux/1 -> [sign_FL]  "FL"
  Demux/2 -> [sign_FR]  "FR"
  Demux/3 -> [sign_RL]  "RL"
  Demux/4 -> [sign_RR]  "RR"
  mode/1 -> "[1-4]"/1
  If Action Subsystem/2(offset) -> Merge1/1
  If Action Subsystem2/2(offset) -> Merge1/3
  If Action Subsystem3/2(offset) -> Merge1/4
  "[1-4]"/1 -> If/1
  If Action Subsystem3/1(sign) -> Merge/4
  If/2 -> If Action Subsystem1/Action
  If Action Subsystem2/1(sign) -> Merge/3
  If Action Subsystem1/1(sign) -> Merge/2
  If Action Subsystem/1(sign) -> Merge/1
  If/1 -> If Action Subsystem/Action
  If/4 -> If Action Subsystem3/Action
  If/3 -> If Action Subsystem2/Action
  If Action Subsystem1/2(offset) -> Merge1/2
  Merge/1 -> Demux/1
  Demux1/4 -> [offest_RR]  "RR"
  Demux1/3 -> [offest_RL]  "RL"
  Demux1/2 -> [offest_FR]  "FR"
  Demux1/1 -> [offest_FL]  "FL"
  Merge1/1 -> Demux1/1
  Multiply/1 -> Sat_FL1/1
  [sign_FL] -> Multiply/1
  [offest_FL] -> Add/1
  [offest_FR] -> Add1/1
  [sign_FR] -> Multiply1/1
  Multiply1/1 -> Sat_FR1/1
  Multiply2/1 -> Sat_RL1/1
  [sign_RL] -> Multiply2/1
  [offest_RL] -> Add2/1
  [offest_RR] -> Add3/1
  [sign_RR] -> Multiply3/1
  Multiply3/1 -> Sat_RR1/1
  Add/1 -> Multiply4/2
  Add1/1 -> Multiply5/2
  Add2/1 -> Multiply6/2
  Add3/1 -> Multiply7/2
  Sat_RL/1 -> Mux/3  "RL_angref_deg"
  Sat_RR/1 -> Mux/4  "RR_angref_deg"
  Sat_FR/1 -> Mux/2  "FR_angref_deg"
  Sat_FL/1 -> Mux/1  "FL_angref_deg"
  Mux/1 -> cmd_out/1
  Multiply4/1 -> Sat_FL/1
  Multiply5/1 -> Sat_FR/1
  Multiply6/1 -> Sat_RL/1
  Multiply7/1 -> Sat_RR/1
  Sat_FL1/1 -> Add/2
  Sat_RL1/1 -> Add2/2
  Sat_FR1/1 -> Add1/2
  Sat_RR1/1 -> Add3/2
  zeroturn_steer_enable/1 -> If Action Subsystem3/1(In1)
  cmd/1 -> Demux2/1
  Demux2/1 -> Multiply/2
  Demux2/2 -> Multiply1/2
  Demux2/3 -> Multiply2/2
  Demux2/4 -> Multiply3/2
  Constant/1 -> Multiply4/1, Multiply7/1, Multiply6/1, Multiply5/1

== system Katex_FullCar_R2017b_V03/Locomotion/Conditioning/Str_LPF ==
  note: s = 2/Ts*(z-1)/(z+1)
  note: H(s) = 1/(tau*s+1)
  note: y(n) = [Ts*{x(n)+x(n-1)}+(2*tau-Ts)*y(n-1)]/(2*tau+Ts)
  note: LPF : tau = 1/(2*pi*fc)
  In : Inport
  fc : Inport  Port=2
  Constant : Constant  Value=Ts  SampleTime=Ts
  Constant1 : Constant  SampleTime=Ts
  Product1 : Product  Inputs=*/  RndMeth=Zero
  Product11 : Product  RndMeth=Zero
  Product2 : Product  Inputs=*/  RndMeth=Zero
  Sum1 : Sum  Inputs=+-  InputSameDT=on  SaturateOnIntegerOverflow=on  OutDataTypeStr=Inherit: Same as first input
  Sum2 : Sum  InputSameDT=on  SaturateOnIntegerOverflow=on  OutDataTypeStr=Inherit: Same as first input
  Sum3 : Sum  InputSameDT=on  SaturateOnIntegerOverflow=on  OutDataTypeStr=Inherit: Same as first input
  Sum4 : Sum  InputSameDT=on  SaturateOnIntegerOverflow=on  OutDataTypeStr=Inherit: Same as first input
  d : UnitDelay  SampleTime=Ts
  d1 : UnitDelay  SampleTime=Ts
  gain : Gain  Gain=Ts  SaturateOnIntegerOverflow=on  OutDataTypeStr=Inherit: Same as input  ParamDataTypeStr=Inherit: Same as input
  gain1 : Gain  Gain=2  SaturateOnIntegerOverflow=on  OutDataTypeStr=Inherit: Same as input  ParamDataTypeStr=Inherit: Same as input
  gain2 : Gain  Gain=2*pi  SaturateOnIntegerOverflow=on  OutDataTypeStr=Inherit: Same as input  ParamDataTypeStr=Inherit: Same as input
  Out : Outport
  wires:
  gain2/1 -> Product2/2
  Constant1/1 -> Product2/1
  Product2/1 -> gain1/1
  Product1/1 -> d/1, Out/1
  Sum4/1 -> Product1/2
  Sum2/1 -> Product1/1
  d/1 -> Product11/2
  gain1/1 -> Sum4/1, Sum1/1
  fc/1 -> gain2/1
  Constant/1 -> Sum4/2, Sum1/2
  Sum1/1 -> Product11/1
  Product11/1 -> Sum2/2
  gain/1 -> Sum2/1
  Sum3/1 -> gain/1
  d1/1 -> Sum3/2
  In/1 -> d1/1, Sum3/1

== system Katex_FullCar_R2017b_V03/Locomotion/Conditioning/Sus_LPF ==
  note: LPF : tau = 1/(2*pi*fc)
  note: y(n) = [Ts*{x(n)+x(n-1)}+(2*tau-Ts)*y(n-1)]/(2*tau+Ts)
  note: H(s) = 1/(tau*s+1)
  note: s = 2/Ts*(z-1)/(z+1)
  In : Inport
  fc : Inport  Port=2
  Constant : Constant  Value=Ts  SampleTime=Ts
  Constant1 : Constant  SampleTime=Ts
  Product1 : Product  Inputs=*/  RndMeth=Zero
  Product11 : Product  RndMeth=Zero
  Product2 : Product  Inputs=*/  RndMeth=Zero
  Sum1 : Sum  Inputs=+-  InputSameDT=on  SaturateOnIntegerOverflow=on  OutDataTypeStr=Inherit: Same as first input
  Sum2 : Sum  InputSameDT=on  SaturateOnIntegerOverflow=on  OutDataTypeStr=Inherit: Same as first input
  Sum3 : Sum  InputSameDT=on  SaturateOnIntegerOverflow=on  OutDataTypeStr=Inherit: Same as first input
  Sum4 : Sum  InputSameDT=on  SaturateOnIntegerOverflow=on  OutDataTypeStr=Inherit: Same as first input
  d : UnitDelay  SampleTime=Ts
  d1 : UnitDelay  SampleTime=Ts
  gain : Gain  Gain=Ts  SaturateOnIntegerOverflow=on  OutDataTypeStr=Inherit: Same as input  ParamDataTypeStr=Inherit: Same as input
  gain1 : Gain  Gain=2  SaturateOnIntegerOverflow=on  OutDataTypeStr=Inherit: Same as input  ParamDataTypeStr=Inherit: Same as input
  gain2 : Gain  Gain=2*pi  SaturateOnIntegerOverflow=on  OutDataTypeStr=Inherit: Same as input  ParamDataTypeStr=Inherit: Same as input
  Out : Outport
  wires:
  In/1 -> Sum3/1, d1/1
  d1/1 -> Sum3/2
  Sum3/1 -> gain/1
  gain/1 -> Sum2/1
  Product11/1 -> Sum2/2
  Sum1/1 -> Product11/1
  Constant/1 -> Sum1/2, Sum4/2
  fc/1 -> gain2/1
  gain1/1 -> Sum1/1, Sum4/1
  d/1 -> Product11/2
  Sum2/1 -> Product1/1
  Sum4/1 -> Product1/2
  Product1/1 -> Out/1, d/1
  Product2/1 -> gain1/1
  Constant1/1 -> Product2/1
  gain2/1 -> Product2/2

== system Katex_FullCar_R2017b_V03/Locomotion/Conditioning/Suspension mode ==
  note: Suspension mode
  note: [0] All synchronize
      | [1] Only FL
      | [2] Only FR
      | [3] Only RL
      | [4] Only RR
  mode : Inport
  cmd : Inport  Port=2
  Constant : Constant
  Demux : Demux
  Demux2 : Demux
  Gain{1..4} (4 alike) : Gain
  If : If  IfExpression=u1==0  ElseIfExpressions=u1==1,u1==2,u1==3,u1==4  ShowElse=off
  If Action Subsystem : Subsystem  TreatAsAtomicUnit=on
  If Action Subsystem1 : Subsystem  TreatAsAtomicUnit=on
  If Action Subsystem2 : Subsystem  TreatAsAtomicUnit=on
  If Action Subsystem3 : Subsystem  TreatAsAtomicUnit=on
  If Action Subsystem4 : Subsystem  TreatAsAtomicUnit=on
  Merge : Merge  Inputs=5
  Multiply{,1..7} (8 alike) : Product
  Mux : Mux
  Scope : Scope  NumInputPorts=4
      settings: ActiveDisplayYMinimum=-1  ActiveDisplayYMaximum=1  DataLoggingVariableName=ScopeData83
  cmd_out : Outport  VectorParamsAs1DForOutWhenUnconnected=off
  wires:
  Gain1/1 -> Multiply/2
  Gain2/1 -> Multiply1/2
  Gain3/1 -> Multiply2/2
  Gain4/1 -> Multiply3/2
  Mux/1 -> cmd_out/1
  Multiply/1 -> Multiply4/2
  Multiply2/1 -> Multiply6/2
  Multiply1/1 -> Multiply5/2
  Multiply3/1 -> Multiply7/2
  If/1 -> If Action Subsystem/Action
  If/2 -> If Action Subsystem1/Action
  If/5 -> If Action Subsystem4/Action
  Demux/4 -> [sign_RR]  "RR"
  Demux/2 -> [sign_FR]  "FR"
  Demux/3 -> [sign_RL]  "RL"
  Merge/1 -> Demux/1
  Demux/1 -> [sign_FL]  "FL"
  If Action Subsystem/1(enable) -> Merge/1
  If Action Subsystem1/1(enable) -> Merge/2
  If Action Subsystem2/1(enable) -> Merge/3
  If/3 -> If Action Subsystem2/Action
  If/4 -> If Action Subsystem3/Action
  If Action Subsystem3/1(enable) -> Merge/4
  If Action Subsystem4/1(enable) -> Merge/5
  mode/1 -> If/1
  [sign_FL] -> Multiply4/1
  [sign_FR] -> Multiply5/1
  [sign_RL] -> Multiply6/1
  [sign_RR] -> Multiply7/1
  Multiply4/1 -> Scope/1, Mux/1  "FL_angref_deg"
  Multiply5/1 -> Scope/2, Mux/2  "FR_angref_deg"
  Multiply6/1 -> Scope/3, Mux/3  "RL_angref_deg"
  Multiply7/1 -> Scope/4, Mux/4  "RR_angref_deg"
  cmd/1 -> Demux2/1
  Demux2/4 -> Gain4/1
  Demux2/3 -> Gain3/1
  Demux2/1 -> Gain1/1
  Demux2/2 -> Gain2/1
  Constant/1 -> Multiply3/1, Multiply2/1, Multiply1/1, Multiply/1

== system Katex_FullCar_R2017b_V03/Locomotion/Initialization/Subsystem ==
  In1 : Inport
  Bus Creator : BusCreator  Inputs=3
  Bus Selector : BusSelector  OutputSignals=FLdrv_tqref_pct,FLstr_tqref_pct,FLsus_tqref_pct
  Out1 : Outport  VectorParamsAs1DForOutWhenUnconnected=off
  wires:
  In1/1 -> Bus Selector/1
  Bus Selector/2 -> Bus Creator/2  "<FLstr_tqref_pct>"
  Bus Selector/1 -> Bus Creator/1  "<FLdrv_tqref_pct>"
  Bus Selector/3 -> Bus Creator/3  "<FLsus_tqref_pct>"
  Bus Creator/1 -> Out1/1

== system Katex_FullCar_R2017b_V03/Locomotion/Initialization/Subsystem1 ==
  In1 : Inport
  Bus Creator : BusCreator  Inputs=3
  Bus Selector : BusSelector  OutputSignals=FRdrv_tqref_pct,FRstr_tqref_pct,FRsus_tqref_pct
  Out1 : Outport  VectorParamsAs1DForOutWhenUnconnected=off
  wires:
  Bus Creator/1 -> Out1/1
  Bus Selector/3 -> Bus Creator/3  "<FRsus_tqref_pct>"
  Bus Selector/1 -> Bus Creator/1  "<FRdrv_tqref_pct>"
  Bus Selector/2 -> Bus Creator/2  "<FRstr_tqref_pct>"
  In1/1 -> Bus Selector/1

== system Katex_FullCar_R2017b_V03/Locomotion/Initialization/Subsystem2 ==
  In1 : Inport
  Bus Creator : BusCreator  Inputs=3
  Bus Selector : BusSelector  OutputSignals=RLdrv_tqref_pct,RLstr_tqref_pct,RLsus_tqref_pct
  Out1 : Outport  VectorParamsAs1DForOutWhenUnconnected=off
  wires:
  In1/1 -> Bus Selector/1
  Bus Selector/2 -> Bus Creator/2  "<RLstr_tqref_pct>"
  Bus Selector/1 -> Bus Creator/1  "<RLdrv_tqref_pct>"
  Bus Selector/3 -> Bus Creator/3  "<RLsus_tqref_pct>"
  Bus Creator/1 -> Out1/1

== system Katex_FullCar_R2017b_V03/Locomotion/Initialization/Subsystem3 ==
  In1 : Inport
  Bus Creator : BusCreator  Inputs=3
  Bus Selector : BusSelector  OutputSignals=RRdrv_tqref_pct,RRstr_tqref_pct,RRsus_tqref_pct
  Out1 : Outport  VectorParamsAs1DForOutWhenUnconnected=off
  wires:
  Bus Creator/1 -> Out1/1
  Bus Selector/3 -> Bus Creator/3  "<RRsus_tqref_pct>"
  Bus Selector/1 -> Bus Creator/1  "<RRdrv_tqref_pct>"
  Bus Selector/2 -> Bus Creator/2  "<RRstr_tqref_pct>"
  In1/1 -> Bus Selector/1

== system Katex_FullCar_R2017b_V03/MuJoCo Interface/FL_Motor_Control/Drv_Driver ==
  In1 : Inport
  In2 : Inport  Port=2
  If1 : If  IfExpression=u1 == 0  ElseIfExpressions=u1 == 1,u1 == 2
  Merge : Merge  Inputs=3
  Position Mode : Subsystem  TreatAsAtomicUnit=on
  Torque Mode : Subsystem  TreatAsAtomicUnit=on
  Velocity Mode : Subsystem  TreatAsAtomicUnit=on
  FL_drive_motor : Outport
  wires:
  If1/1 -> Position Mode/Action
  If1/2 -> Velocity Mode/Action
  If1/3 -> Torque Mode/Action
  Position Mode/1(Out1) -> Merge/1
  Torque Mode/1(controlgain) -> Merge/3
  In1/1 -> If1/1
  Velocity Mode/1(controlgain) -> Merge/2
  In2/1 -> Torque Mode/1(In1), Velocity Mode/1(In1), Position Mode/1(In1)
  Merge/1 -> FL_drive_motor/1
  [drv_motor_zeta] -> Velocity Mode/2(In2)
  [drv_motor_freq] -> Velocity Mode/3(In3)
  [FLdrv_angvel_rads] -> Velocity Mode/4(In4)
  [wheel_radius] -> Velocity Mode/5(In5)

== system Katex_FullCar_R2017b_V03/MuJoCo Interface/FL_Motor_Control/Str_Driver ==
  In1 : Inport
  In2 : Inport  Port=2
  If1 : If  IfExpression=u1 == 0  ElseIfExpressions=u1 == 1,u1 == 2
  Merge : Merge  Inputs=3
  Position Mode : Subsystem  TreatAsAtomicUnit=on
  Torque Mode : Subsystem  TreatAsAtomicUnit=on
  Velocity Mode : Subsystem  TreatAsAtomicUnit=on
  FL_steer_motor : Outport
  wires:
  Merge/1 -> FL_steer_motor/1
  In2/1 -> Position Mode/1(In1), Velocity Mode/1(In1), Torque Mode/1(In1)
  Velocity Mode/1(Out1) -> Merge/2
  In1/1 -> If1/1
  Torque Mode/1(controlgain) -> Merge/3
  Position Mode/1(Out1) -> Merge/1
  If1/3 -> Torque Mode/Action
  If1/2 -> Velocity Mode/Action
  If1/1 -> Position Mode/Action
  [str_motor_zeta] -> Position Mode/2(In2)
  [str_motor_freq] -> Position Mode/3(In3)
  [FLstr_ang_rad] -> Position Mode/4(In4)
  [FLstr_angvel_rads] -> Position Mode/5(velocity_rad_s)

== system Katex_FullCar_R2017b_V03/MuJoCo Interface/FL_Motor_Control/Sus_Driver ==
  In1 : Inport
  In2 : Inport  Port=2
  If1 : If  IfExpression=u1 == 0  ElseIfExpressions=u1 == 1,u1 == 2
  Merge : Merge  Inputs=3
  Position Mode : Subsystem  TreatAsAtomicUnit=on
  Torque Mode : Subsystem  TreatAsAtomicUnit=on
  Velocity Mode : Subsystem  TreatAsAtomicUnit=on
  FL_sus_motor : Outport
  wires:
  If1/1 -> Position Mode/Action
  If1/2 -> Velocity Mode/Action
  If1/3 -> Torque Mode/Action
  Position Mode/1(Out1) -> Merge/1
  In1/1 -> If1/1
  Velocity Mode/1(Out1) -> Merge/2
  Merge/1 -> FL_sus_motor/1
  [sus_motor_zeta] -> Position Mode/2(In2)
  [sus_motor_freq] -> Position Mode/3(In3)
  [FLsus_ang_rad] -> Position Mode/4(In4)
  [FLsus_angvel_rads] -> Position Mode/5(velocity_rad_s)
  Torque Mode/1(controlgain) -> Merge/3
  In2/1 -> Torque Mode/1(In1), Velocity Mode/1(In1), Position Mode/1(In1)

== system Katex_FullCar_R2017b_V03/MuJoCo Interface/FR_Motor_Control/Drv_Driver ==
  In1 : Inport
  In2 : Inport  Port=2
  If1 : If  IfExpression=u1 == 0  ElseIfExpressions=u1 == 1,u1 == 2
  Merge : Merge  Inputs=3
  Position Mode : Subsystem  TreatAsAtomicUnit=on
  Torque Mode : Subsystem  TreatAsAtomicUnit=on
  Velocity Mode : Subsystem  TreatAsAtomicUnit=on
  FR_drive_motor : Outport
  wires:
  [wheel_radius] -> Velocity Mode/5(In5)
  [FRdrv_angvel_rads] -> Velocity Mode/4(In4)
  [drv_motor_freq] -> Velocity Mode/3(In3)
  [drv_motor_zeta] -> Velocity Mode/2(In2)
  Merge/1 -> FR_drive_motor/1
  In2/1 -> Position Mode/1(In1), Velocity Mode/1(In1), Torque Mode/1(In1)
  Velocity Mode/1(controlgain) -> Merge/2
  In1/1 -> If1/1
  Torque Mode/1(controlgain) -> Merge/3
  Position Mode/1(Out1) -> Merge/1
  If1/3 -> Torque Mode/Action
  If1/2 -> Velocity Mode/Action
  If1/1 -> Position Mode/Action

== system Katex_FullCar_R2017b_V03/MuJoCo Interface/FR_Motor_Control/Str_Driver ==
  In1 : Inport
  In2 : Inport  Port=2
  If1 : If  IfExpression=u1 == 0  ElseIfExpressions=u1 == 1,u1 == 2
  Merge : Merge  Inputs=3
  Position Mode : Subsystem  TreatAsAtomicUnit=on
  Torque Mode : Subsystem  TreatAsAtomicUnit=on
  Velocity Mode : Subsystem  TreatAsAtomicUnit=on
  FR_steer_motor : Outport
  wires:
  [FRstr_angvel_rads] -> Position Mode/5(velocity_rad_s)
  [FRstr_ang_rad] -> Position Mode/4(In4)
  [str_motor_freq] -> Position Mode/3(In3)
  [str_motor_zeta] -> Position Mode/2(In2)
  If1/1 -> Position Mode/Action
  If1/2 -> Velocity Mode/Action
  If1/3 -> Torque Mode/Action
  Position Mode/1(Out1) -> Merge/1
  Torque Mode/1(controlgain) -> Merge/3
  In1/1 -> If1/1
  Velocity Mode/1(Out1) -> Merge/2
  In2/1 -> Torque Mode/1(In1), Velocity Mode/1(In1), Position Mode/1(In1)
  Merge/1 -> FR_steer_motor/1

== system Katex_FullCar_R2017b_V03/MuJoCo Interface/FR_Motor_Control/Sus_Driver ==
  In1 : Inport
  In2 : Inport  Port=2
  If1 : If  IfExpression=u1 == 0  ElseIfExpressions=u1 == 1,u1 == 2
  Merge : Merge  Inputs=3
  Position Mode : Subsystem  TreatAsAtomicUnit=on
  Torque Mode : Subsystem  TreatAsAtomicUnit=on
  Velocity Mode : Subsystem  TreatAsAtomicUnit=on
  FR_sus_motor : Outport
  wires:
  [FRsus_angvel_rads] -> Position Mode/5(velocity_rad_s)
  [FRsus_ang_rad] -> Position Mode/4(In4)
  [sus_motor_freq] -> Position Mode/3(In3)
  [sus_motor_zeta] -> Position Mode/2(In2)
  Merge/1 -> FR_sus_motor/1
  In2/1 -> Position Mode/1(In1), Velocity Mode/1(In1), Torque Mode/1(In1)
  Velocity Mode/1(Out1) -> Merge/2
  In1/1 -> If1/1
  Torque Mode/1(controlgain) -> Merge/3
  Position Mode/1(Out1) -> Merge/1
  If1/3 -> Torque Mode/Action
  If1/2 -> Velocity Mode/Action
  If1/1 -> Position Mode/Action

== system Katex_FullCar_R2017b_V03/MuJoCo Interface/RL_Motor_Control/Drv_Driver ==
  In1 : Inport
  In2 : Inport  Port=2
  If1 : If  IfExpression=u1 == 0  ElseIfExpressions=u1 == 1,u1 == 2
  Merge : Merge  Inputs=3
  Position Mode : Subsystem  TreatAsAtomicUnit=on
  Torque Mode : Subsystem  TreatAsAtomicUnit=on
  Velocity Mode : Subsystem  TreatAsAtomicUnit=on
  RL_drive_motor : Outport
  wires:
  [wheel_radius] -> Velocity Mode/5(In5)
  [RLdrv_angvel_rads] -> Velocity Mode/4(In4)
  [drv_motor_freq] -> Velocity Mode/3(In3)
  [drv_motor_zeta] -> Velocity Mode/2(In2)
  Merge/1 -> RL_drive_motor/1
  In2/1 -> Position Mode/1(In1), Velocity Mode/1(In1), Torque Mode/1(In1)
  Velocity Mode/1(controlgain) -> Merge/2
  In1/1 -> If1/1
  Torque Mode/1(controlgain) -> Merge/3
  Position Mode/1(Out1) -> Merge/1
  If1/3 -> Torque Mode/Action
  If1/2 -> Velocity Mode/Action
  If1/1 -> Position Mode/Action

== system Katex_FullCar_R2017b_V03/MuJoCo Interface/RL_Motor_Control/Str_Driver ==
  In1 : Inport
  In2 : Inport  Port=2
  If1 : If  IfExpression=u1 == 0  ElseIfExpressions=u1 == 1,u1 == 2
  Merge : Merge  Inputs=3
  Position Mode : Subsystem  TreatAsAtomicUnit=on
  Torque Mode : Subsystem  TreatAsAtomicUnit=on
  Velocity Mode : Subsystem  TreatAsAtomicUnit=on
  RL_steer_motor : Outport
  wires:
  [RLstr_angvel_rads] -> Position Mode/5(velocity_rad_s)
  [RLstr_ang_rad] -> Position Mode/4(In4)
  [str_motor_freq] -> Position Mode/3(In3)
  [str_motor_zeta] -> Position Mode/2(In2)
  If1/1 -> Position Mode/Action
  If1/2 -> Velocity Mode/Action
  If1/3 -> Torque Mode/Action
  Position Mode/1(Out1) -> Merge/1
  Torque Mode/1(controlgain) -> Merge/3
  In1/1 -> If1/1
  Velocity Mode/1(Out1) -> Merge/2
  In2/1 -> Torque Mode/1(In1), Velocity Mode/1(In1), Position Mode/1(In1)
  Merge/1 -> RL_steer_motor/1

== system Katex_FullCar_R2017b_V03/MuJoCo Interface/RL_Motor_Control/Sus_Driver ==
  In1 : Inport
  In2 : Inport  Port=2
  If1 : If  IfExpression=u1 == 0  ElseIfExpressions=u1 == 1,u1 == 2
  Merge : Merge  Inputs=3
  Position Mode : Subsystem  TreatAsAtomicUnit=on
  Torque Mode : Subsystem  TreatAsAtomicUnit=on
  Velocity Mode : Subsystem  TreatAsAtomicUnit=on
  RL_sus_motor : Outport
  wires:
  [RLsus_angvel_rads] -> Position Mode/5(velocity_rad_s)
  [RLsus_ang_rad] -> Position Mode/4(In4)
  [sus_motor_freq] -> Position Mode/3(In3)
  [sus_motor_zeta] -> Position Mode/2(In2)
  Merge/1 -> RL_sus_motor/1
  In2/1 -> Position Mode/1(In1), Velocity Mode/1(In1), Torque Mode/1(In1)
  Velocity Mode/1(Out1) -> Merge/2
  In1/1 -> If1/1
  Torque Mode/1(controlgain) -> Merge/3
  Position Mode/1(Out1) -> Merge/1
  If1/3 -> Torque Mode/Action
  If1/2 -> Velocity Mode/Action
  If1/1 -> Position Mode/Action
